simulink model "Comunicacao_Simulink_R2018b"  (R2018b)
settings: Solver=VariableStepAuto  StartTime=0.0  StopTime=8  RelTol=1e-3
libraries: dspsrcs4 x2, commsynccomp2 x1, simulink x1, commfilt2 x1, commutil2 x1
settings Model: Creator=rafae  LastModifiedBy=rafae

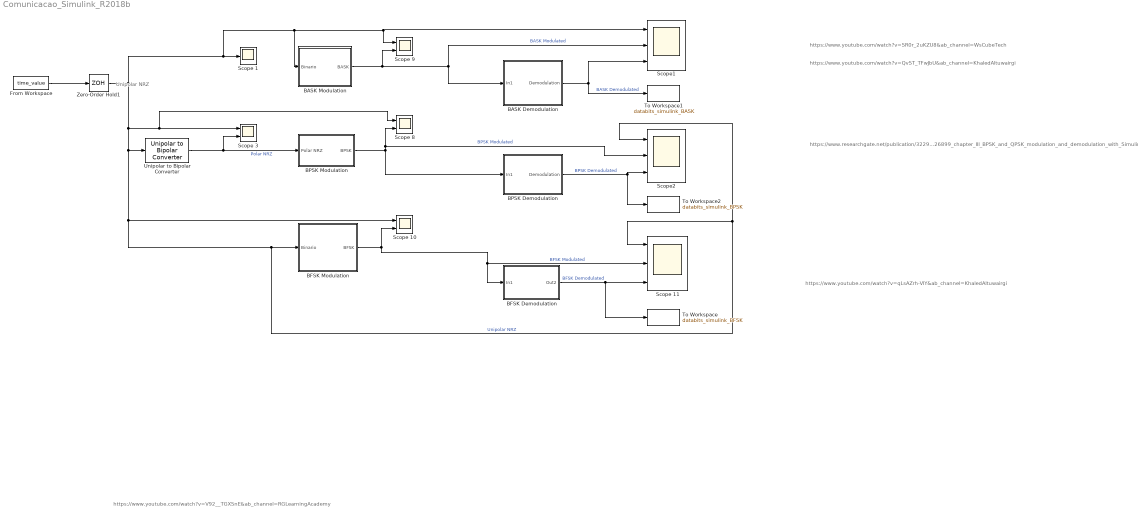
== system Comunicacao_Simulink_R2018b ==
  note: Unipolar NRZ
  note: https://www.researchgate.net/publication/322926899_chapter_III_BPSK_and_QPSK_modulation_and_demodulation_with_Simulink
  note: https://www.youtube.com/watch?v=SR0r_2uKZU8&ab_channel=WsCubeTech
  note: https://www.youtube.com/watch?v=qLsAZrh-VIY&ab_channel=KhaledAltuwairgi
  note: https://www.youtube.com/watch?v=V92__TGXSnE&ab_channel=RGLearningAcademy
  note: https://www.youtube.com/watch?v=QvST_TFwJbU&ab_channel=KhaledAltuwairgi
  BASK Demodulation : Subsystem
  BASK Modulation : Subsystem
  BFSK Demodulation : Subsystem
  BFSK Modulation : Subsystem
  BPSK Demodulation : Subsystem
  BPSK Modulation : Subsystem
  From Workspace : FromWorkspace  VariableName=time_value  SampleTime=0
  Scope 1 : Scope
  Scope {3,8..10} (4 alike) : Scope  NumInputPorts=2
  Scope 11 : Scope  NumInputPorts=3
  Scope1 : Scope  NumInputPorts=3
  Scope2 : Scope  NumInputPorts=3
  To Workspace : ToWorkspace  VariableName=databits_simulink_BFSK  SaveFormat=Timeseries  SampleTime=-1
  To Workspace1 : ToWorkspace  VariableName=databits_simulink_BASK  SaveFormat=Timeseries  SampleTime=-1
  To Workspace2 : ToWorkspace  VariableName=databits_simulink_BPSK  SaveFormat=Timeseries  SampleTime=-1
  Unipolar to Bipolar Converter : commutil2/Unipolar to Bipolar Converter  M=2  polarity=Positive  dataType=Inherit via internal rule
      settings: SourceProductName=Communications Toolbox
  Zero-Order Hold1 : ZeroOrderHold  SampleTime=-1
  wires:
  Zero-Order Hold1/1 -> BASK Modulation/1(Binario), Scope 9/1, Scope1/1, Scope 1/1, Scope 3/1, Scope 8/1, Scope 10/1, Scope2/1, Scope 11/1, BFSK Modulation/1(Binario), Unipolar to Bipolar Converter/1  "Unipolar NRZ"
  Unipolar to Bipolar Converter/1 -> Scope 3/2, BPSK Modulation/1(Polar NRZ)  "Polar NRZ"
  From Workspace/1 -> Zero-Order Hold1/1
  BASK Modulation/1(BASK) -> Scope 9/2, BASK Demodulation/1(In1), Scope1/2  "BASK Modulated"
  BPSK Modulation/1(BPSK) -> BPSK Demodulation/1(In1), Scope2/2, Scope 8/2  "BPSK Modulated"
  BFSK Modulation/1(BFSK) -> BFSK Demodulation/1(In1), Scope 11/2, Scope 10/2  "BFSK Modulated"
  BASK Demodulation/1(Demodulation) -> Scope1/3, To Workspace1/1  "BASK Demodulated"
  BPSK Demodulation/1(Demodulation) -> Scope2/3, To Workspace2/1  "BPSK Demodulated"
  BFSK Demodulation/1(Out2) -> To Workspace/1, Scope 11/3  "BFSK Demodulated"

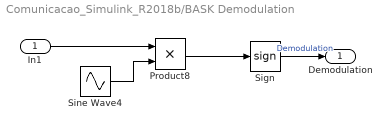
== system Comunicacao_Simulink_R2018b/BASK Demodulation ==
  In1 : Inport
  Product8 : Product
  Sign : Signum
  Sine Wave4 : Sin  Frequency=2*pi*2  SampleTime=0
  Demodulation : Outport
  wires:
  Sine Wave4/1 -> Product8/2
  Product8/1 -> Sign/1
  Sign/1 -> Demodulation/1  "Demodulation"
  In1/1 -> Product8/1

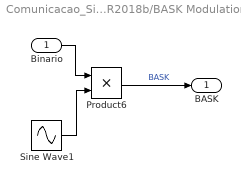
== system Comunicacao_Simulink_R2018b/BASK Modulation ==
  Binario : Inport
  Product6 : Product
  Sine Wave1 : Sin  Frequency=2*pi*2  SampleTime=0
  BASK : Outport
  wires:
  Sine Wave1/1 -> Product6/2
  Binario/1 -> Product6/1
  Product6/1 -> BASK/1  "BASK"

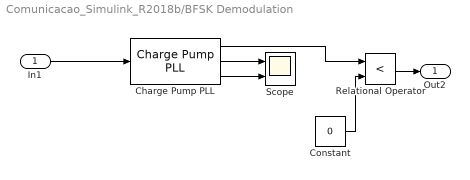
== system Comunicacao_Simulink_R2018b/BFSK Demodulation ==
  In1 : Inport
  Charge Pump PLL : commsynccomp2/Charge Pump PLL  Fn=[2*pi*1]  Fd=[1 2*pi*1]  Kvco=4  Fc=10  Ph=0  Ac=1
      settings: SourceProductName=Communications Toolbox  SourceProductBaseCode=CM
  Constant : Constant  Value=0
  Relational Operator : RelationalOperator  Operator=<  OutDataTypeStr=boolean  RndMeth=Simplest
  Scope : Scope  NumInputPorts=2
  Out2 : Outport
  wires:
  Charge Pump PLL/2 -> Scope/1
  Constant/1 -> Relational Operator/2
  Charge Pump PLL/3 -> Scope/2
  Charge Pump PLL/1 -> Relational Operator/1
  In1/1 -> Charge Pump PLL/1
  Relational Operator/1 -> Out2/1

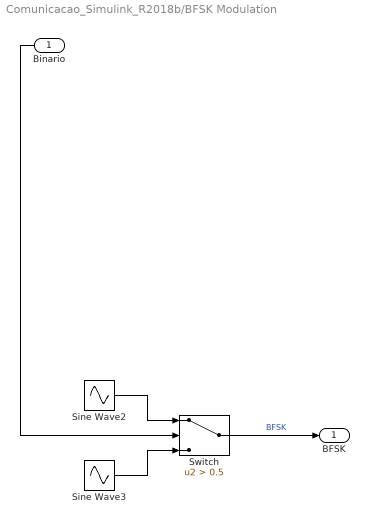
== system Comunicacao_Simulink_R2018b/BFSK Modulation ==
  Binario : Inport
  Sine Wave2 : Sin  Frequency=2*pi*4  SampleTime=0
  Sine Wave3 : Sin  Frequency=2*pi*12  SampleTime=0
  Switch : Switch  Criteria=u2 > Threshold  Threshold=0.5
  BFSK : Outport
  wires:
  Binario/1 -> Switch/2
  Sine Wave3/1 -> Switch/3
  Sine Wave2/1 -> Switch/1
  Switch/1 -> BFSK/1  "BFSK"

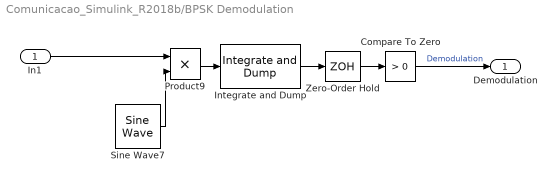
== system Comunicacao_Simulink_R2018b/BPSK Demodulation ==
  In1 : Inport
  Compare To Zero : simulink/Logic and Bit Operations/Compare To Zero  relop=>  OutDataTypeStr=boolean
  Integrate and Dump : commfilt2/Integrate and Dump  obssamples=100  offsetsamples=0  nodump=on  roundingMode=Floor  overflowMode=off  outputDataTypeStr=Inherit: Same as accumulator  outputLastDataTypeStr=Inherit: Same as accumulator
      settings: SourceProductName=Communications Toolbox
  Product9 : Product
  Sine Wave7 : dspsrcs4/Sine Wave  Amplitude=1  Frequency=5  Phase=0  SampleMode=Discrete  OutComplex=Real  CompMethod=Trigonometric fcn  TableSize=Speed  SampleTime=1/1000  SamplesPerFrame=1  ResetState=Restart at time zero  OutputFrames=off  dataType=double  wordLen=16  udDataType=sfix(16)  fracBitsMode=Best precision  numFracBits=15  OutDataTypeStr=double  LastOutDataTypeStr=double
  Zero-Order Hold : ZeroOrderHold  SampleTime=-1
  Demodulation : Outport
  wires:
  Integrate and Dump/1 -> Zero-Order Hold/1
  In1/1 -> Product9/1
  Sine Wave7/1 -> Product9/2
  Zero-Order Hold/1 -> Compare To Zero/1
  Compare To Zero/1 -> Demodulation/1  "Demodulation"
  Product9/1 -> Integrate and Dump/1

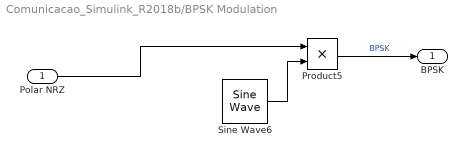
== system Comunicacao_Simulink_R2018b/BPSK Modulation ==
  Polar NRZ : Inport
  Product5 : Product
  Sine Wave6 : dspsrcs4/Sine Wave  Amplitude=1  Frequency=5  Phase=0  SampleMode=Discrete  OutComplex=Real  CompMethod=Trigonometric fcn  TableSize=Speed  SampleTime=1/1000  SamplesPerFrame=1  ResetState=Restart at time zero  OutputFrames=off  dataType=double  wordLen=16  udDataType=sfix(16)  fracBitsMode=Best precision  numFracBits=15  OutDataTypeStr=double  LastOutDataTypeStr=double
  BPSK : Outport
  wires:
  Sine Wave6/1 -> Product5/2
  Polar NRZ/1 -> Product5/1
  Product5/1 -> BPSK/1  "BPSK"
